simulink model "SafetyCriticalLQR"  (R2020b)
settings: Solver=VariableStepAuto  StartTime=0.0  StopTime=tf_upperbound  RelTol=1e-7  AbsTol=1e-7
PreLoadFcn:
  | SafetyCriticalLQRParams
values from neighbouring files (symbols this model uses):
  A = 0    [RCBFSim.mat]    (also in SafetyCriticalLQRParams.m)
  B = 1    [RCBFSim.mat]    (also in SafetyCriticalLQRParams.m)
  beta = 0.9    [RCBFSim.m]    (also in RCBFSim.mat; SafetyCriticalLQRParams.m = 0.1)
  C = 1    [RCBFSim.mat]    (also in SafetyCriticalLQRParams.m)
  D = 0    [RCBFSim.mat]    (also in SafetyCriticalLQRParams.m)
  eta = 2    [RCBFSim.mat]    (also in SafetyCriticalLQRParams.m)
  filterCase = 4    [RCBFSim.m]    (also in RCBFSim.mat; SafetyCriticalLQRParams.m = 1)
  gamma = 1    [RCBFSim.mat]    (also in SafetyCriticalLQRParams.m)
  K = 0.4472135955    [RCBFSim.mat]
  P = 2.2360679775    [RCBFSim.mat]
  Ref = 0    [RCBFSim.mat]    (also in SafetyCriticalLQRParams.m)
  x0 = 0.5    [RCBFSim.mat]    (also in SafetyCriticalLQRParams.m)
libraries: simulink x1
settings Model: Creator=Jyot Buch  LastModifiedBy=Jyot Buch

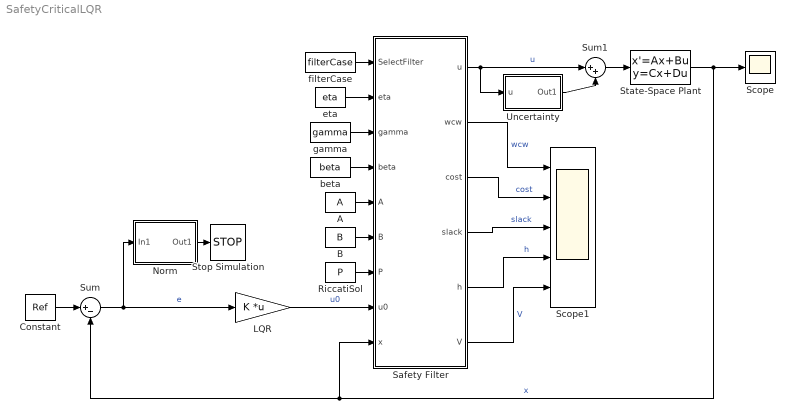
== system SafetyCriticalLQR ==
  A : Constant  Value=A
  B : Constant  Value=B
  Constant : Constant  Value=Ref
  LQR : Gain  Gain=K  Multiplication=Matrix(K*u) (u vector)
  Norm : Subsystem
  RiccatiSol : Constant  Value=P
  Safety Filter : MATLAB Function  TreatAsAtomicUnit=on
  Scope : Scope
  Scope1 : Scope  NumInputPorts=5
  State-Space Plant : StateSpace  A=A  B=B  C=C  D=D  InitialCondition=x0
  Stop Simulation : Stop
  Sum : Sum  Inputs=|+-
  Sum1 : Sum  Inputs=|++
  Uncertainty : Subsystem
  beta : Constant  Value=beta
  eta : Constant  Value=eta
  filterCase : Constant  Value=filterCase
  gamma : Constant  Value=gamma
  wires:
  State-Space Plant/1 -> Safety Filter/9(x), Sum/2, Scope/1  "x"
  Constant/1 -> Sum/1
  Sum/1 -> LQR/1, Norm/1(In1)  "e"
  LQR/1 -> Safety Filter/8(u0)  "u0"
  Safety Filter/1(u) -> Sum1/1, Uncertainty/1(u)  "u"
  filterCase/1 -> Safety Filter/1(SelectFilter)
  RiccatiSol/1 -> Safety Filter/7(P)
  Safety Filter/5(h) -> Scope1/4  "h"
  Safety Filter/6(V) -> Scope1/5  "V"
  Norm/1(Out1) -> Stop Simulation/1
  eta/1 -> Safety Filter/2(eta)
  gamma/1 -> Safety Filter/3(gamma)
  Safety Filter/4(slack) -> Scope1/3  "slack"
  A/1 -> Safety Filter/5(A)
  B/1 -> Safety Filter/6(B)
  beta/1 -> Safety Filter/4(beta)
  Safety Filter/2(wcw) -> Scope1/1  "wcw"
  Safety Filter/3(cost) -> Scope1/2  "cost"
  Sum1/1 -> State-Space Plant/1
  Uncertainty/1(Out1) -> Sum1/2

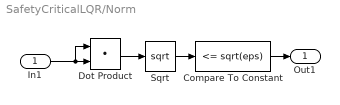
== system SafetyCriticalLQR/Norm ==
  In1 : Inport
  Compare To Constant : simulink/Logic and Bit Operations/Compare To Constant  relop=<=  const=sqrt(eps)  OutDataTypeStr=boolean
  Dot Product : DotProduct  InputSameDT=on  OutDataTypeStr=Inherit: Inherit via internal rule
  Sqrt : Sqrt  SaturateOnIntegerOverflow=on
  Out1 : Outport
  wires:
  In1/1 -> Dot Product/1, Dot Product/2
  Dot Product/1 -> Sqrt/1
  Sqrt/1 -> Compare To Constant/1
  Compare To Constant/1 -> Out1/1

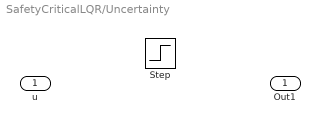
== system SafetyCriticalLQR/Uncertainty ==
  u : Inport
  Step : Step  SampleTime=0
  Out1 : Outport

== matlab function SafetyCriticalLQR/Safety Filter ==
  data: u output; wcw output; cost output; SelectFilter input; eta input; gamma input; beta input; A input; B input; P input; u0 input; slack output; x input; h output; V output
function [u,wcw,cost,slack,h,V] = fcn(SelectFilter,eta,gamma,beta,A,B,P,u0,x)
%% FCN
% Compute h and V
p = -1;
h = -x + 1;
V = x'*P*x;
slack = 0;
cost = 0;

% Select filter based on the specified case
switch SelectFilter
    case 1
        % Nominal LQR
        u = u0;
        wcw = 0;
        
    case 2
        % CBF Only
        [u,cost] = CBFQP(eta,h,u0,x);
        wcw = 0;
        
    case 3
        % CLF-CBF
        [u,cost,slack] = CLFCBFQP(eta,gamma,h,V,A,B,P,u0,x);
        wcw = 0;
        
    case 4
        % Robust CBF with LinProgTick
        [u,cost] = RobustCBFQPLinProgTick(eta,beta,h,u0,x);        
        wcw = -beta*sign(p)*abs(u);
        
    otherwise
        % Openloop
        u = u0*0;
        wcw = 0;
end
end

%% CBFQP
function [u,cost] = CBFQP(eta,h,u0,x)
% Inequality Safety Constraints for QP
% Aineq'*u <= bineq
Aineq = -1;
bineq = x + eta*h;

% Solve QP
SolveQPCase = 1;
switch SolveQPCase
    case 1
        % Numerical Solution
        H = 1;
        f = -u0;
        opt = optimoptions('quadprog','Algorithm','active-set','Display','off');
        [u,cost] = quadprog(H,f,Aineq,bineq,[],[],[],[],u0,opt);
        cost = cost + 0.5*(u0'*u0);
        
    case 2
        % Explicit Solution
        rho = -bineq+Aineq*u0;
        if rho<=0
            zopt = 0;
        else
            zopt = -rho*Aineq/Aineq^2;
        end
        u = zopt+u0;
        cost = 0.5*(zopt'*zopt);
end
end

%% CLFCBFQP
function [u,cost,slack] = CLFCBFQP(eta,gamma,h,V,A,B,P,u0,x)
% Slack variable penalty
m = 1;

% Inequality Constraints for QP
% Safety: hdot >= -alpha*h
Aineq1 = [-1 0];
bineq1 = x + eta*h;

% Stability: Vdot <= -beta*V
Aineq2 = [2*x'*P*B -1];
bineq2 = -x'*(A'*P + P*A)*x - gamma*V;

% Aineq'*[u;delta] <= bineq
Aineq = [Aineq1; Aineq2];
bineq = [bineq1; bineq2];

% Solve QP
H = diag([1, m]);
opt = optimoptions('quadprog','Algorithm','active-set','Display','off');
[sol,cost] = quadprog(H,[],Aineq,bineq,[],[],[],[],[u0;0],opt);

% Read outputs
u = sol(1);
slack = sol(2);
end

%% RobustCBFQPLinProgTick
function [u,cost] = RobustCBFQPLinProgTick(eta,beta,h,u0,x)
% Inequality Constraints for QP
% Aineq'*u <= bineq
p = -1;

% Solve QP
if (-x-u0+beta*sign(p)*abs(u0)) >= -eta*h
    % Choose nominal control
    u = u0;
    cost = 0.5*(u0'*u0);
else
    Aineq = [-2*p*(1 - sign(p)*beta) +2*p*(sign(p)*beta + 1); -1 0;0 -1];
    bineq = [x + eta*h; 0; 0];
    H = [1 -1;-1 1];
    f = [-u0 +u0];
    opt = optimoptions('quadprog','Algorithm','active-set','Display','off');
    [uStar,cost] = quadprog(H,f,Aineq,bineq,[],[],[],[],[u0;u0]*0,opt);
    cost = cost + 0.5*(u0'*u0);
    
    % up and un
    up = uStar(1);
    un = uStar(2);
    
    % Output
    u = up - un;
end
end
